simulink model "cdnlink_lb_wide_15a"  (Simulink 8.5)
settings: Solver=ode45  StartTime=0.0  StopTime=10.0  RelTol=1e-3
undefined symbols (not defined in the file): des, gcbh
(part 3 of 3)

== matlab function R1/Routing Table ==
  data: y output double; timer input double; lb_algo input double; router_sel input double; x output double; load1 input double; load3 input double; load5 input double; load7 input double; d3 input double; d5 input double; d7 input double; reply input double; source input double; content_time input double; packet_id input double; dest input double; hop_count input double; router_id input double
function [y, x]  = fcn(timer, lb_algo, router_sel, load1, load3, load5, ...
    load7, d3, d5, d7, reply, source, content_time, ...
    packet_id, dest, hop_count, router_id)

y = nan;
x = hop_count + 1;
this_cluster = 1;
algorithm = lb_algo;
% Algorithm:
%
% 1. Random               RAND
% 2. Round Robin          RR
% 3. Least Loaded         LL
% 4. Two Random Choices   2RC
%

switch reply
    
    case 1 % Reply
        
        switch packet_id
            case 1
                if timer < 5
                    y = 2;
                    %hop_count = hop_count + 1;
                    %x = hop_count;
                else
                    switch router_sel
                        case 1
                            %%% Selected as: 1. Regular router
                            %%%              2. SoR
                            
                            switch algorithm
                                
                                case 3 % DNS-based Least Loaded
                                    
                                    switch dest
                                        case this_cluster
                                            y = 2;
                                        case 7
                                            y = 7;
                                        case 3
                                            y = 3;
                                        otherwise
                                            y = 5;
                                    end;
                            end; % Algorithm on Regular Router
                            
                        otherwise % Router_sel = 2 --> SoR
                            
                            switch algorithm
                                
                                case 0 % No LB algorithm. Local server only.
                                    y = 2;
                                    
                                case 1 % RAND Algorithm
                                    
                                    if source == 3
                                        x_dest = [2 5 7];
                                        y = x_dest(randi(length(x_dest)));
                                    else
                                        if source == 5
                                            x_dest = [2 3 7];
                                            y = x_dest(randi(length(x_dest)));
                                        else
                                            if source == 7
                                                x_dest = [2 3 5 ];
                                                y = x_dest(randi(length(x_dest)));
                                            else
                                                x_dest = [2 3 5 7];
                                                y = x_dest(randi(length(x_dest)));
                                            end;
                                        end;
                                    end;
                                    
                                case 2 % RR Algo
                                    
                                case 3 % LL Algorithm with CET (hard coded)
                                    
                                    %x_source = [1 3 5 7];
                                    
                                    if content_time >= 0.1121
                                        
                                        if router_id == 3 || router_id == 1
                                            if load1 == min([load1 load5])
                                                y = 2;
                                            else
                                                y = 5;
                                            end;
                                        else
                                            y = 2;
                                        end;
                                        
                                    else
                                        if router_id == 3
                                            if load1 == min([load1 load5 load7])
                                                y = 2;
                                            else
                                                if load5 == min([load1 load5 load7])
                                                    y = 5;
                                                else
                                                    y = 7;
                                                end;
                                            end;
                                        else
                                            if router_id == 5
                                                if load1 == min([load1 load3 load7])
                                                    y = 2;
                                                else
                                                    if load3 == min([load1 load3 load7])
                                                        y = 3;
                                                    else
                                                        y = 7;
                                                    end;
                                                end;
                                            else
                                                if router_id == 7
                                                    if load1 == min([load1 load5 load3])
                                                        y = 2;
                                                    else
                                                        if load5 == min([load1 load5 load3])
                                                            y = 5;
                                                        else
                                                            y = 3;
                                                        end;
                                                    end;
                                                    
                                                else
                                                    if load1 == min([load1 load3 load5 load7])
                                                        y = 2;
                                                    else
                                                        if load3 == min([load1 load3 load5 load7])
                                                            y = 3;
                                                        else
                                                            if load5 == min([load1 load3 load5 load7])
                                                                y = 5;
                                                            else
                                                                y = 7;
                                                            end;
                                                        end;
                                                    end;
                                                end;
                                            end;
                                        end;
                                    end;
                                    
                                case 4 % SoR LL Algorithm based on waiting time
                                    
                                    %x_source = [1 3 5 7];
                                    %content_time = 0.1
                                    
                                    %if content_time >= 0.1121
                                    
                                    if router_id == 3
                                        if d1 == min([d1 d5 d7])
                                            y = 2;
                                        else
                                            if d5 == min([d1 d5 d7])
                                                y = 5;
                                            else
                                                y = 7;
                                            end;
                                        end;
                                    else
                                        if router_id == 5
                                            if d1 == min([d1 d3 d7])
                                                y = 2;
                                            else
                                                if d5 == min([d1 d5 d7])
                                                    y = 5;
                                                else
                                                    y = 7;
                                                end;
                                            end;
                                        else
                                            if router_id == 7
                                                if d1 == min([d1 d3 d5])
                                                    y = 2;
                                                else
                                                    if d3 == min([d1 d3 d5])
                                                        y = 3;
                                                    else
                                                        y = 5;
                                                    end;
                                                end;
                                            else
                                                if d1 == min([d1 d3 d5 d7])
                                                    y = 2;
                                                else
                                                    if d3 == min([d1 d3 d5 d7])
                                                        y = 3;
                                                    else
                                                        if d5 == min([d1 d3 d5 d7])
                                                            y = 5;
                                                        else
                                                            y = 7;
                                                        end;
                                                    end;
                                                end;
                                            end;
                                        end;
                                    end;
                                    
                                case 5 % SoR LL Algorithm with CET
                                    
                                otherwise
                            end % Algorithm
                    end; % router_sel
                end;
                
            case 2 % packet_id == 2
                y = 5;
                
            case 4
                y = 2;
                
            case 5
                y = 2;
                
            case 6 
                if dest == 3
                    y = 3;
                    if dest == 7
                        y = 7;
                    else
                        y = 5;
                    end;
                end;

                
%             case 8
%                 switch dest
%                     case 1
%                         y = 2;
%                     case 3
%                         y = 3;
%                     case 5
%                         y = 5;
%                     case 7
%                         y = 7;
%                     otherwise
%                         y = 15;
%                 end;
                
            otherwise
                y = 15;
        end; % packet id on Reply = 1
        
    case 2 % Reply = 2
        
        switch packet_id
            case {1 2}
                switch source
                    case this_cluster
                        y = 1;
                    case 3
                        y = 3;
                    case 7
                        y = 7;
                    otherwise
                        y = 5;
                end;
                
            case 4 % packet id = 4
                y = 5;
            
            otherwise
                y = 15;
        end; %packet id
        
    otherwise
        y = 15;
end; % Reply

== matlab function R3/MATLAB Function ==
  data: timer input double; lb_algo input double; router_sel input double; x output double; load1 input double; load3 input double; load5 input double; d1 input double; d5 input double; reply input double; source input double; content_time input double; y output double; packet_id input double; dest input double; hop_count input double; router_id input double
function [x, y]  = fcn(timer, lb_algo, router_sel, ...
    load1, load3, load5, d1, d5, reply, source, ...
    content_time, packet_id, dest, hop_count, router_id)

%%%%%
% CDNlink Routing Table
% For Reg Router and SoR
% by. Erwin Harahap (c) 2015
% Keio Univ. Japan.
%%%%%%

y = nan;
x = hop_count + 1;
this_cluster = 3;
algorithm = lb_algo;

% Algorithm:
%
% 1. Random               RAND
% 2. Round Robin          RR
% 3. Least Loaded         LL
% 4. Two Random Choices   2RC
%
%
%

if reply == 2
    if packet_id == 1 || packet_id == 2
        if source == this_cluster
            y = 1;
        else
            if source == 1 || source == 7
                y = 11;
            else
                y = 5;
            end;
        end;
    else
        if packet_id == 4
            y = 5;
            %             if packet_id == 8
            %                 y = 11;
            %             end;
        end;
    end;
else
    if reply == 1
        if packet_id == 1;
            
            if timer < 5
                y = 2;
            else
                
                if hop_count >=20
                    y = 2;
                else
                    if router_sel == 1
                        %%% 1. Regular Router
                        %%% 2. SoR
                        if algorithm == 3
                            if dest == this_cluster
                                y = 2;
                            else
                                if dest == 1 || dest == 7
                                    y = 1;
                                else
                                    y = 5;
                                end;
                            end;
                        end;
                    else
                        if router_sel == 2
                            %%% 1. Regular Router
                            %%% 2. SoR
                            
                            if algorithm == 0
                                y = 2;
                            else
                                
                                if algorithm == 1
                                    
                                    %%% RAND Alg
                                    
                                    if source == 1
                                        x_dest = [2 5];
                                        y = x_dest(randi(length(x_dest)));
                                    else
                                        if source == 5
                                            x_dest = [2 11];
                                            y = x_dest(randi(length(x_dest)));
                                        else
                                            x_dest = [2 5 11];
                                            y = x_dest(randi(length(x_dest)));
                                        end;
                                    end;
                                else
                                    
                                    %%% LL Algorithm
                                    
                                    if algorithm == 3
                                        
                                        if content_time >= 0.1121
                                            
                                            if router_id == 3 || router_id == 1
                                                if load1 == min([load1 load5])
                                                    y = 2;
                                                else
                                                    y = 5;
                                                end;
                                            else
                                                y = 2;
                                            end;
                                            
                                        else
                                            if router_id == 3
                                                if load1 == min([load1 load5])
                                                    y = 2;
                                                else
                                                    y = 5;
                                                end;
                                            else
                                                if router_id == 5
                                                    if load1 == min([load1 load3])
                                                        y = 2;
                                                    else
                                                        y = 3;
                                                    end;
                                                else
                                                    if load1 == min([load1 load3 load5])
                                                        y = 2;
                                                    else
                                                        if load3 == min([load1 load3 load5])
                                                            y = 3;
                                                        else
                                                            y = 5;
                                                        end;
                                                    end;
                                                end;
                                            end;
                                        end;
                                    end;
                                    %%% End A
                                end;
                            end;
                        end;
                    end;
                end;
            end;
        else
            
            if packet_id == 2
                y = 5;
            else
                
                if packet_id == 4
                    y = 2;
                else
                    
                    if packet_id == 5
                        y = 2;
                        
                    else
                        if packet_id == 6
                            if dest == 1
                                y = 11;
                            else
                                if dest == 5
                                    y = 5;
                                else
                                    y = 13;
                                end;
                            end;
                        else
                            
                            
                            %                     else
                            %
                            %                         if packet_id == 8
                            %                             y = 2;
                            %                         else
                            
                            y = 13;
                        end;
                    end;
                end;
            end;
        end;
    else
        y = 12;
    end;
end;
